simulink model "Lab5"  (R2022b)
settings: Solver=VariableStepAuto  StartTime=0.0  StopTime=10.0  MaxStep=1e-3  RelTol=1e-3
libraries: simulink x3
settings Model: Creator=LOQ  LastModifiedBy=LOQ
settings OptimizationCC: ReuseModelBlockBuffer=on
settings RTWCC: GPUComputeCapability=5.0
settings ConfigComp: CovBoundaryAbsTol=1.0e-5

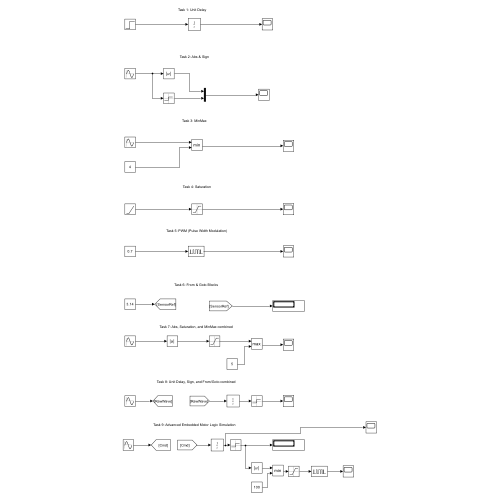
[thumbnail: Simulink's stored preview of the top-level diagram]
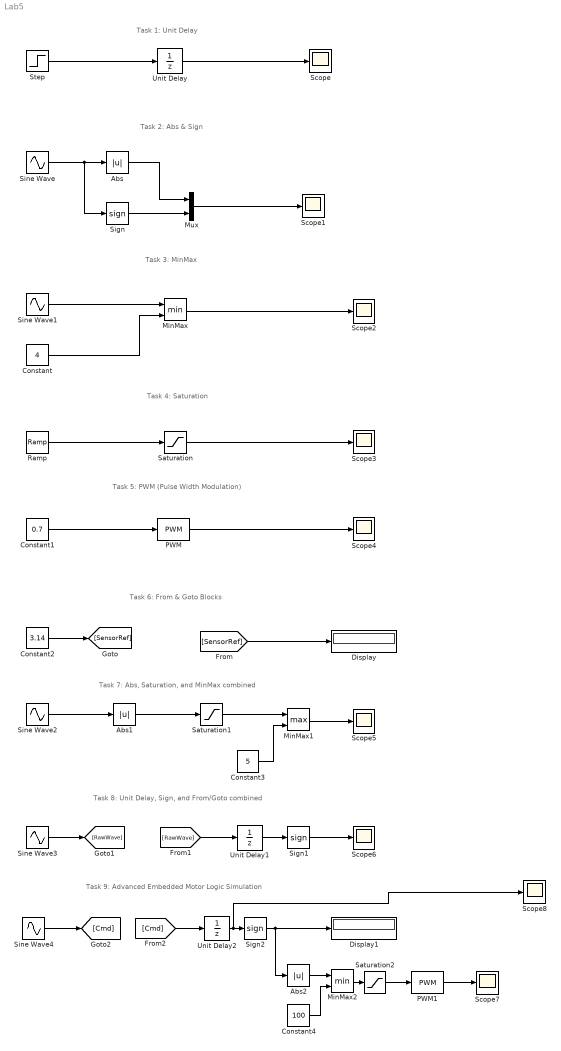
== system Lab5 ==
  note: Task 9: Advanced Embedded Motor Logic Simulation
  note: Task 8: Unit Delay, Sign, and From/Goto combined
  note: Task 7: Abs, Saturation, and MinMax combined
  note: Task 6: From & Goto Blocks
  note: Task 5: PWM (Pulse Width Modulation)
  note: Task 4: Saturation
  note: Task 3: MinMax
  note: Task 2: Abs & Sign
  note: Task 1: Unit Delay
  Abs : Abs  SaturateOnIntegerOverflow=off
  Abs1 : Abs  SaturateOnIntegerOverflow=off
  Abs2 : Abs  SaturateOnIntegerOverflow=off
  Constant : Constant  Value=4
  Constant1 : Constant  Value=0.7
  Constant2 : Constant  Value=3.14
  Constant3 : Constant  Value=5
  Constant4 : Constant  Value=100
  Display : Display
  Display1 : Display
  MinMax : MinMax  Inputs=2
  MinMax1 : MinMax  Function=max  Inputs=2
  MinMax2 : MinMax  Inputs=2
  Mux : Mux  Inputs=2
  PWM : simulink/Discontinuities/PWM  DisableCoverage=on  Period=1  InitialDelay=0  DisallowZeroDutyCycle=off  RunAtFixedTimeIntervals=off  SampleTime=0.1
  PWM1 : simulink/Discontinuities/PWM  DisableCoverage=on  Period=1  InitialDelay=0  DisallowZeroDutyCycle=off  RunAtFixedTimeIntervals=off  SampleTime=0.1
  Ramp : simulink/Sources/Ramp  slope=2  start=0  InitialOutput=0
  Saturation : Saturate  UpperLimit=8  LowerLimit=2
  Saturation1 : Saturate  UpperLimit=15  LowerLimit=0
  Saturation2 : Saturate
  Scope{,1..8} (9 alike) : Scope
  Sign : Signum
  Sign1 : Signum
  Sign2 : Signum
  Sine Wave : Sin  Amplitude=5  SampleTime=0
  Sine Wave1 : Sin  Amplitude=10  SampleTime=0
  Sine Wave2 : Sin  Amplitude=20  SampleTime=0
  Sine Wave3 : Sin  Amplitude=150  SampleTime=0
  Sine Wave4 : Sin  Amplitude=150  SampleTime=0
  Step : Step  Time=2  After=10  SampleTime=0
  Unit Delay : UnitDelay  HasFrameUpgradeWarning=on
  Unit Delay1 : UnitDelay  SampleTime=0.5  HasFrameUpgradeWarning=on
  Unit Delay2 : UnitDelay  HasFrameUpgradeWarning=on
  wires:
  Step/1 -> Unit Delay/1
  Unit Delay/1 -> Scope/1
  Sine Wave/1 -> Sign/1, Abs/1
  Mux/1 -> Scope1/1
  Abs/1 -> Mux/1
  Sign/1 -> Mux/2
  Sine Wave1/1 -> MinMax/1
  Constant/1 -> MinMax/2
  MinMax/1 -> Scope2/1
  Ramp/1 -> Saturation/1
  Saturation/1 -> Scope3/1
  Constant1/1 -> PWM/1
  PWM/1 -> Scope4/1
  Constant2/1 -> [SensorRef]
  [SensorRef] -> Display/1
  Sine Wave2/1 -> Abs1/1
  Abs1/1 -> Saturation1/1
  Saturation1/1 -> MinMax1/1
  Constant3/1 -> MinMax1/2
  MinMax1/1 -> Scope5/1
  Sine Wave3/1 -> [RawWave]
  [RawWave] -> Unit Delay1/1
  Unit Delay1/1 -> Sign1/1
  Sign1/1 -> Scope6/1
  Sine Wave4/1 -> [Cmd]
  Unit Delay2/1 -> Scope8/1, Sign2/1
  [Cmd] -> Unit Delay2/1
  Sign2/1 -> Display1/1, Abs2/1
  Abs2/1 -> MinMax2/1
  Constant4/1 -> MinMax2/2
  MinMax2/1 -> Saturation2/1
  Saturation2/1 -> PWM1/1
  PWM1/1 -> Scope7/1
